simulink model "Simulacion_Estrategias"  (R2016a)
settings: Solver=VariableStepAuto  StartTime=0.0  StopTime=5  RelTol=1e-3
undefined symbols (not defined in the file): AL, BL, CL, DL, Kes_PC, Kest_LQR, Ki_PC, u10, u20, u30, x10, x20, x30, xini1
libraries: cstblocks x12
settings Model: Creator=Lenovo  LastModifiedBy=Lenovo

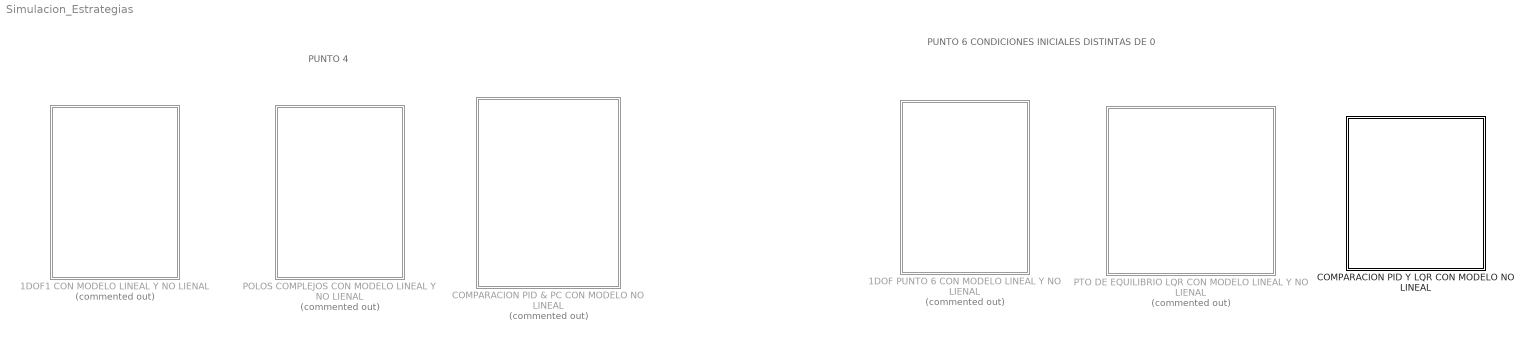
== system Simulacion_Estrategias ==
  note: PUNTO 6 CONDICIONES INICIALES DISTINTAS DE 0
  note: PUNTO 4
  1DOF PUNTO 6 CON MODELO LINEAL Y NO LIENAL : Subsystem  Commented=on
  1DOF1 CON MODELO LINEAL Y NO LIENAL : Subsystem  Commented=on
  COMPARACION PID & PC CON MODELO NO LINEAL : Subsystem  Commented=on
  COMPARACION PID Y LQR CON MODELO NO LINEAL : Subsystem
  "POLOS COMPLEJOS CON MODELO LINEAL Y NO LIENAL " : Subsystem  Commented=on
  PTO DE EQUILIBRIO LQR CON MODELO LINEAL Y NO LIENAL : Subsystem  Commented=on

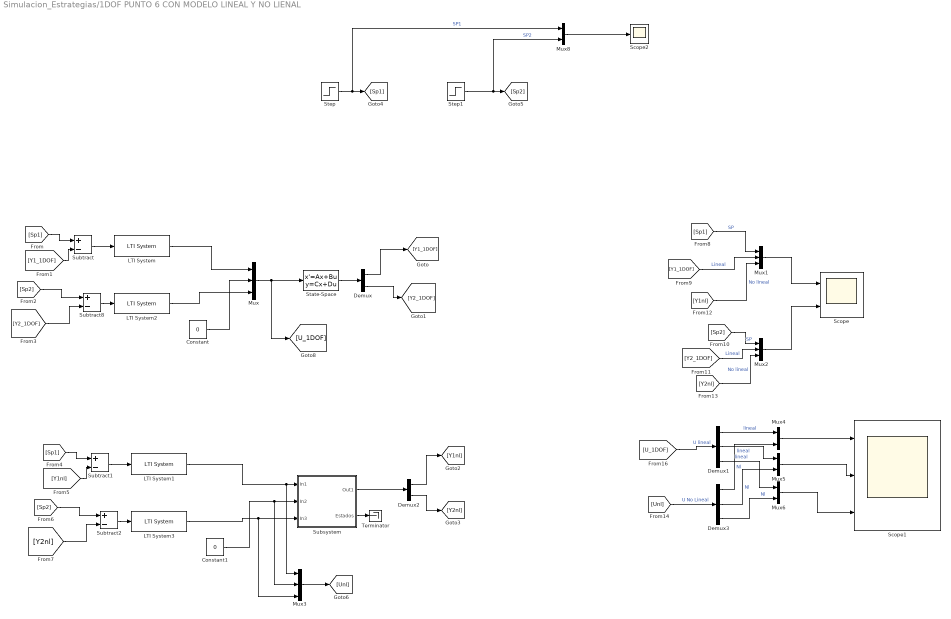
== system Simulacion_Estrategias/1DOF PUNTO 6 CON MODELO LINEAL Y NO LIENAL ==
  Constant : Constant  Value=0
  Constant1 : Constant  Value=0
  Demux : Demux  Outputs=2
  Demux1 : Demux  Outputs=3
  Demux2 : Demux  Outputs=2
  Demux3 : Demux  Outputs=3
  LTI System : cstblocks/LTI System  sys=C11  IC=[]
  LTI System1 : cstblocks/LTI System  sys=C11  IC=[]
  LTI System2 : cstblocks/LTI System  sys=C23  IC=[]
  LTI System3 : cstblocks/LTI System  sys=C23  IC=[]
  Mux{,1..3} (4 alike) : Mux  Inputs=3
  Mux{4..6,8} (4 alike) : Mux  Inputs=2
  Scope : Scope  NumInputPorts=2
  Scope1 : Scope  NumInputPorts=3
  Scope2 : Scope
  State-Space : StateSpace  A=AL  B=BL  C=CL  D=DL  X0=xini1
  Step : Step  Time=0  After=0  SampleTime=0
  Step1 : Step  Time=0  After=0  SampleTime=0
  Subsystem : Subsystem
  Subtract{,1..2,8} (4 alike) : Sum  Inputs=+-
  Terminator : Terminator
  wires:
  Constant1/1 -> Subsystem/2(In2), Mux3/2
  LTI System3/1 -> Subsystem/3(In3), Mux3/3
  LTI System1/1 -> Subsystem/1(In1), Mux3/1
  LTI System2/1 -> Mux/3
  Constant/1 -> Mux/2
  LTI System/1 -> Mux/1
  [Y1nl] -> Subtract1/2
  [Sp1] -> Subtract1/1
  [Sp2] -> Subtract2/1
  Subtract2/1 -> LTI System3/1
  Subtract1/1 -> LTI System1/1
  [Y2nl] -> Subtract2/2
  Demux3/3 -> Mux6/2  "Nl"
  Demux3/2 -> Mux5/2  "Nl"
  Demux3/1 -> Mux4/2  "Nl"
  Demux1/3 -> Mux6/1  "lineal"
  Demux1/2 -> Mux5/1  "lineal"
  Demux1/1 -> Mux4/1  "lineal"
  Mux6/1 -> Scope1/3
  [Y2nl] -> Mux2/3  "No lineal"
  [Y1_1DOF] -> Mux1/2  "Lineal"
  [U_1DOF] -> Demux1/1  "U lineal"
  Mux5/1 -> Scope1/2
  [Unl] -> Demux3/1  "U No Lineal"
  Demux2/1 -> [Y1nl]
  [Y1nl] -> Mux1/3  "No lineal"
  [Sp1] -> Mux1/1  "SP"
  Mux2/1 -> Scope/2
  Mux4/1 -> Scope1/1
  [Sp2] -> Mux2/1  "SP"
  Subsystem/1(Out1) -> Demux2/1
  Demux2/2 -> [Y2nl]
  Mux1/1 -> Scope/1
  [Y2_1DOF] -> Mux2/2  "Lineal"
  State-Space/1 -> Demux/1
  [Y2_1DOF] -> Subtract8/2
  Subtract/1 -> LTI System/1
  Subtract8/1 -> LTI System2/1
  [Sp2] -> Subtract8/1
  Mux/1 -> [U_1DOF], State-Space/1
  Demux/2 -> [Y2_1DOF]
  Demux/1 -> [Y1_1DOF]
  [Sp1] -> Subtract/1
  [Y1_1DOF] -> Subtract/2
  Mux3/1 -> [Unl]
  Subsystem/2(Estados) -> Terminator/1
  Step/1 -> Mux8/1, [Sp1]  "SP1"
  Step1/1 -> Mux8/2, [Sp2]  "SP2"
  Mux8/1 -> Scope2/1

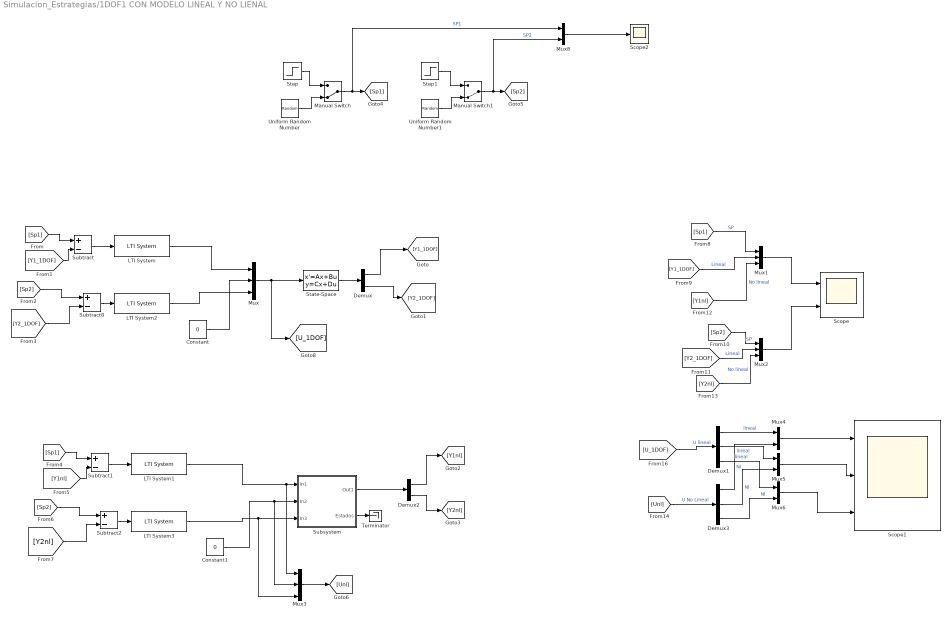
== system Simulacion_Estrategias/1DOF1 CON MODELO LINEAL Y NO LIENAL ==
  Constant : Constant  Value=0
  Constant1 : Constant  Value=0
  Demux : Demux  Outputs=2
  Demux1 : Demux  Outputs=3
  Demux2 : Demux  Outputs=2
  Demux3 : Demux  Outputs=3
  LTI System : cstblocks/LTI System  sys=C11  IC=[]
  LTI System1 : cstblocks/LTI System  sys=C11  IC=[]
  LTI System2 : cstblocks/LTI System  sys=C23  IC=[]
  LTI System3 : cstblocks/LTI System  sys=C23  IC=[]
  Manual Switch : ManualSwitch  CurrentSetting=0
  Manual Switch1 : ManualSwitch  CurrentSetting=0
  Mux{,1..3} (4 alike) : Mux  Inputs=3
  Mux{4..6,8} (4 alike) : Mux  Inputs=2
  Scope : Scope  NumInputPorts=2
  Scope1 : Scope  NumInputPorts=3
  Scope2 : Scope
  State-Space : StateSpace  A=AL  B=BL  C=CL  D=DL
  Step : Step  Time=0  SampleTime=0
  Step1 : Step  Time=0  After=0  SampleTime=0
  Subsystem : Subsystem
  Subtract{,1..2,8} (4 alike) : Sum  Inputs=+-
  Terminator : Terminator
  Uniform Random Number : UniformRandomNumber  Minimum=-0-5  Maximum=0.5  SampleTime=4
  Uniform Random Number1 : UniformRandomNumber  Minimum=-0.5  Maximum=0.5  SampleTime=7
  wires:
  Mux8/1 -> Scope2/1
  Manual Switch1/1 -> [Sp2], Mux8/2  "SP2"
  Step1/1 -> Manual Switch1/1
  Uniform Random Number/1 -> Manual Switch/2
  Manual Switch/1 -> [Sp1], Mux8/1  "SP1"
  Step/1 -> Manual Switch/1
  Uniform Random Number1/1 -> Manual Switch1/2
  Subsystem/2(Estados) -> Terminator/1
  Mux3/1 -> [Unl]
  [Y1_1DOF] -> Subtract/2
  [Sp1] -> Subtract/1
  Demux/1 -> [Y1_1DOF]
  Demux/2 -> [Y2_1DOF]
  Mux/1 -> State-Space/1, [U_1DOF]
  [Sp2] -> Subtract8/1
  Subtract8/1 -> LTI System2/1
  Subtract/1 -> LTI System/1
  [Y2_1DOF] -> Subtract8/2
  State-Space/1 -> Demux/1
  [Y2_1DOF] -> Mux2/2  "Lineal"
  Mux1/1 -> Scope/1
  Demux2/2 -> [Y2nl]
  Subsystem/1(Out1) -> Demux2/1
  [Sp2] -> Mux2/1  "SP"
  Mux4/1 -> Scope1/1
  Mux2/1 -> Scope/2
  [Sp1] -> Mux1/1  "SP"
  [Y1nl] -> Mux1/3  "No lineal"
  Demux2/1 -> [Y1nl]
  [Unl] -> Demux3/1  "U No Lineal"
  Mux5/1 -> Scope1/2
  [U_1DOF] -> Demux1/1  "U lineal"
  [Y1_1DOF] -> Mux1/2  "Lineal"
  [Y2nl] -> Mux2/3  "No lineal"
  Mux6/1 -> Scope1/3
  Demux1/1 -> Mux4/1  "lineal"
  Demux1/2 -> Mux5/1  "lineal"
  Demux1/3 -> Mux6/1  "lineal"
  Demux3/1 -> Mux4/2  "Nl"
  Demux3/2 -> Mux5/2  "Nl"
  Demux3/3 -> Mux6/2  "Nl"
  [Y2nl] -> Subtract2/2
  Subtract1/1 -> LTI System1/1
  Subtract2/1 -> LTI System3/1
  [Sp2] -> Subtract2/1
  [Sp1] -> Subtract1/1
  [Y1nl] -> Subtract1/2
  LTI System/1 -> Mux/1
  Constant/1 -> Mux/2
  LTI System2/1 -> Mux/3
  LTI System1/1 -> Mux3/1, Subsystem/1(In1)
  LTI System3/1 -> Mux3/3, Subsystem/3(In3)
  Constant1/1 -> Mux3/2, Subsystem/2(In2)

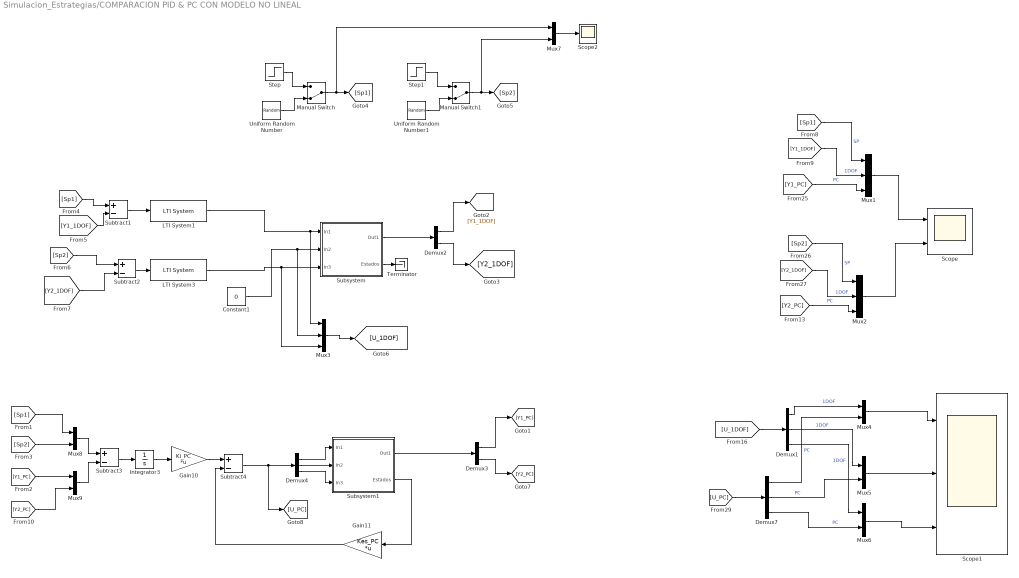
== system Simulacion_Estrategias/COMPARACION PID & PC CON MODELO NO LINEAL ==
  Constant1 : Constant  Value=0
  Demux1 : Demux  Outputs=3
  Demux2 : Demux  Outputs=2
  Demux3 : Demux  Outputs=2
  Demux4 : Demux  Outputs=3
  Demux7 : Demux  Outputs=3
  Gain10 : Gain  Gain=Ki_PC  Multiplication=Matrix(K*u)
  Gain11 : Gain  Gain=Kes_PC  Multiplication=Matrix(K*u)
  Integrator3 : Integrator
  LTI System1 : cstblocks/LTI System  sys=C11  IC=[]
  LTI System3 : cstblocks/LTI System  sys=C23  IC=[]
  Manual Switch : ManualSwitch  CurrentSetting=0
  Manual Switch1 : ManualSwitch  CurrentSetting=0
  Mux1 : Mux  Inputs=3
  Mux2 : Mux  Inputs=3
  Mux3 : Mux  Inputs=3
  Mux{4..9} (6 alike) : Mux  Inputs=2
  Scope : Scope  NumInputPorts=2
  Scope1 : Scope  NumInputPorts=3
  Scope2 : Scope
  Step : Step  Time=0  After=0  SampleTime=0
  Step1 : Step  Time=0  SampleTime=0
  Subsystem : Subsystem
  Subsystem1 : Subsystem
  Subtract{1..4} (4 alike) : Sum  Inputs=+-
  Terminator : Terminator
  Uniform Random Number : UniformRandomNumber  Minimum=-0.5  Maximum=0.5  SampleTime=6
  Uniform Random Number1 : UniformRandomNumber  Minimum=-0.5  Maximum=0.5  SampleTime=9
  wires:
  Uniform Random Number1/1 -> Manual Switch1/2
  Mux7/1 -> Scope2/1
  Manual Switch1/1 -> [Sp2], Mux7/2
  Uniform Random Number/1 -> Manual Switch/2
  Manual Switch/1 -> [Sp1], Mux7/1
  Step/1 -> Manual Switch/1
  Step1/1 -> Manual Switch1/1
  Mux5/1 -> Scope1/2
  Mux6/1 -> Scope1/3
  [Sp1] -> Mux1/1  "SP"
  [Y1_1DOF] -> Mux1/2  "1DOF"
  Mux1/1 -> Scope/1
  [U_PC] -> Demux7/1
  [U_1DOF] -> Demux1/1
  Demux1/3 -> Mux6/1  "1DOF"
  [Y2_1DOF] -> Mux2/2  "1DOF"
  [Y1_PC] -> Mux1/3  "PC"
  Demux1/2 -> Mux5/1  "1DOF"
  Mux4/1 -> Scope1/1
  Demux1/1 -> Mux4/1  "1DOF"
  Mux2/1 -> Scope/2
  [Sp2] -> Mux2/1  "SP"
  [Y2_PC] -> Mux2/3  "PC"
  Demux7/1 -> Mux4/2  "PC"
  Demux7/2 -> Mux5/2  "PC"
  Demux7/3 -> Mux6/2  "PC"
  LTI System1/1 -> Mux3/1, Subsystem/1(In1)
  Subtract2/1 -> LTI System3/1
  [Sp1] -> Subtract1/1
  [Y1_1DOF] -> Subtract1/2
  [Y2_1DOF] -> Subtract2/2
  Subsystem/2(Estados) -> Terminator/1
  [Sp2] -> Subtract2/1
  Demux2/1 -> [Y1_1DOF]
  Mux3/1 -> [U_1DOF]
  Subsystem/1(Out1) -> Demux2/1
  Subtract1/1 -> LTI System1/1
  Demux2/2 -> [Y2_1DOF]
  Constant1/1 -> Mux3/2, Subsystem/2(In2)
  LTI System3/1 -> Mux3/3, Subsystem/3(In3)
  Subsystem1/2(Estados) -> Gain11/1
  Demux4/2 -> Subsystem1/2(In2)
  Subsystem1/1(Out1) -> Demux3/1
  Demux4/1 -> Subsystem1/1(In1)
  [Y1_PC] -> Mux9/1
  Mux8/1 -> Subtract3/1
  Demux4/3 -> Subsystem1/3(In3)
  Subtract3/1 -> Integrator3/1
  Gain10/1 -> Subtract4/1
  [Sp2] -> Mux8/2
  Gain11/1 -> Subtract4/2
  Integrator3/1 -> Gain10/1
  Subtract4/1 -> [U_PC], Demux4/1
  [Sp1] -> Mux8/1
  [Y2_PC] -> Mux9/2
  Demux3/2 -> [Y2_PC]
  Mux9/1 -> Subtract3/2
  Demux3/1 -> [Y1_PC]

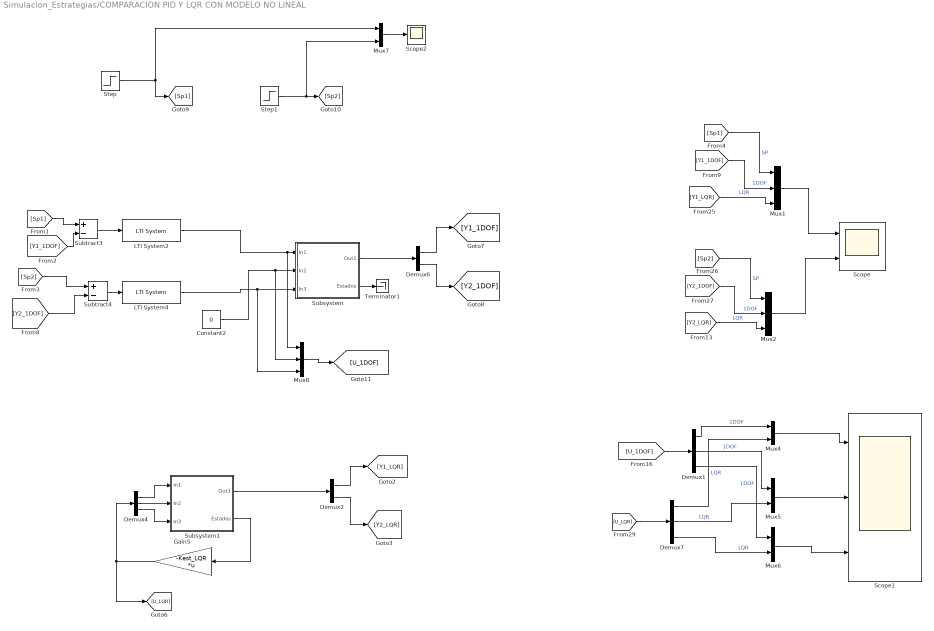
== system Simulacion_Estrategias/COMPARACION PID Y LQR CON MODELO NO LINEAL ==
  Constant2 : Constant  Value=0
  Demux1 : Demux  Outputs=3
  Demux2 : Demux  Outputs=2
  Demux4 : Demux  Outputs=3
  Demux6 : Demux  Outputs=2
  Demux7 : Demux  Outputs=3
  Gain5 : Gain  Gain=-Kest_LQR  Multiplication=Matrix(K*u)
  LTI System2 : cstblocks/LTI System  sys=C11  IC=[]
  LTI System4 : cstblocks/LTI System  sys=C23  IC=[]
  Mux1 : Mux  Inputs=3
  Mux2 : Mux  Inputs=3
  Mux{4..7} (4 alike) : Mux  Inputs=2
  Mux8 : Mux  Inputs=3
  Scope : Scope  NumInputPorts=2
  Scope1 : Scope  NumInputPorts=3
  Scope2 : Scope
  Step : Step  Time=0  After=0  SampleTime=0
  Step1 : Step  Time=0  After=0  SampleTime=0
  Subsystem : Subsystem
  Subsystem1 : Subsystem
  Subtract3 : Sum  Inputs=+-
  Subtract4 : Sum  Inputs=+-
  Terminator1 : Terminator
  wires:
  Step/1 -> [Sp1], Mux7/1
  Mux7/1 -> Scope2/1
  Step1/1 -> [Sp2], Mux7/2
  Demux4/1 -> Subsystem1/1(In1)
  Subsystem1/2(Estados) -> Gain5/1
  Subsystem1/1(Out1) -> Demux2/1
  Gain5/1 -> Demux4/1, [U_LQR]
  Demux4/2 -> Subsystem1/2(In2)
  Demux2/1 -> [Y1_LQR]
  Demux2/2 -> [Y2_LQR]
  Demux4/3 -> Subsystem1/3(In3)
  LTI System4/1 -> Subsystem/3(In3), Mux8/3
  Subtract3/1 -> LTI System2/1
  Constant2/1 -> Subsystem/2(In2), Mux8/2
  Demux6/2 -> [Y2_1DOF]
  Subsystem/1(Out1) -> Demux6/1
  Mux8/1 -> [U_1DOF]
  [Sp1] -> Subtract3/1
  Subsystem/2(Estados) -> Terminator1/1
  [Y2_1DOF] -> Subtract4/2
  Demux6/1 -> [Y1_1DOF]
  [Y1_1DOF] -> Subtract3/2
  Subtract4/1 -> LTI System4/1
  [Sp2] -> Subtract4/1
  LTI System2/1 -> Subsystem/1(In1), Mux8/1
  [Sp2] -> Mux2/1  "SP"
  Mux2/1 -> Scope/2
  Demux7/1 -> Mux4/2  "LQR"
  [U_LQR] -> Demux7/1
  Demux1/3 -> Mux6/1  "1DOF"
  [Y2_LQR] -> Mux2/3  "LQR"
  Demux7/2 -> Mux5/2  "LQR"
  Mux4/1 -> Scope1/1
  [Y2_1DOF] -> Mux2/2  "1DOF"
  [Y1_LQR] -> Mux1/3  "LQR"
  Demux1/2 -> Mux5/1  "1DOF"
  [U_1DOF] -> Demux1/1
  Demux1/1 -> Mux4/1  "1DOF"
  Mux1/1 -> Scope/1
  Mux5/1 -> Scope1/2
  Mux6/1 -> Scope1/3
  Demux7/3 -> Mux6/2  "LQR"
  [Y1_1DOF] -> Mux1/2  "1DOF"
  [Sp1] -> Mux1/1  "SP"

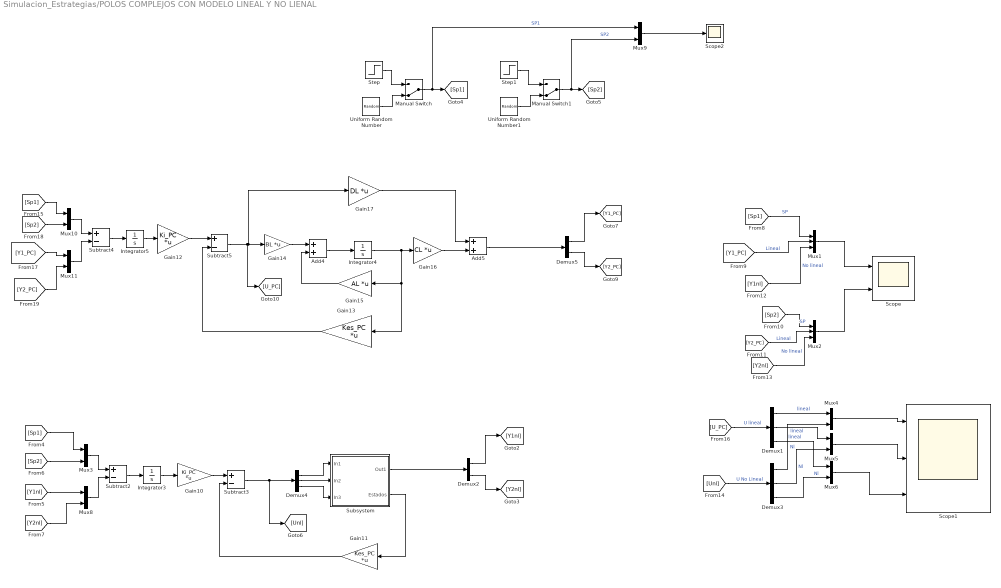
== system Simulacion_Estrategias/POLOS COMPLEJOS CON MODELO LINEAL Y NO LIENAL  ==
  Add4 : Sum
  Add5 : Sum
  Demux1 : Demux  Outputs=3
  Demux2 : Demux  Outputs=2
  Demux3 : Demux  Outputs=3
  Demux4 : Demux  Outputs=3
  Demux5 : Demux  Outputs=2
  Gain10 : Gain  Gain=Ki_PC  Multiplication=Matrix(K*u)
  Gain11 : Gain  Gain=Kes_PC  Multiplication=Matrix(K*u)
  Gain12 : Gain  Gain=Ki_PC  Multiplication=Matrix(K*u)
  Gain13 : Gain  Gain=Kes_PC  Multiplication=Matrix(K*u)
  Gain14 : Gain  Gain=BL  Multiplication=Matrix(K*u)
  Gain15 : Gain  Gain=AL  Multiplication=Matrix(K*u)
  Gain16 : Gain  Gain=CL  Multiplication=Matrix(K*u)
  Gain17 : Gain  Gain=DL  Multiplication=Matrix(K*u)
  Integrator3 : Integrator
  Integrator4 : Integrator
  Integrator5 : Integrator
  Manual Switch : ManualSwitch  CurrentSetting=0
  Manual Switch1 : ManualSwitch  CurrentSetting=0
  Mux1 : Mux  Inputs=3
  Mux{3..6,8..11} (8 alike) : Mux  Inputs=2
  Mux2 : Mux  Inputs=3
  Scope : Scope  NumInputPorts=2
  Scope1 : Scope  NumInputPorts=3
  Scope2 : Scope
  Step : Step  Time=0  SampleTime=0
  Step1 : Step  Time=0  After=0  SampleTime=0
  Subsystem : Subsystem
  Subtract{2..5} (4 alike) : Sum  Inputs=+-
  Uniform Random Number : UniformRandomNumber  Minimum=-0.5  Maximum=0.5  SampleTime=6
  Uniform Random Number1 : UniformRandomNumber  Minimum=-0.5  Maximum=0.5  SampleTime=10
  wires:
  Gain11/1 -> Subtract3/2
  [Y2_PC] -> Mux2/2  "Lineal"
  Mux1/1 -> Scope/1
  Demux2/2 -> [Y2nl]
  [Sp1] -> Mux3/1
  Mux3/1 -> Subtract2/1
  [Sp2] -> Mux2/1  "SP"
  Demux4/2 -> Subsystem/2(In2)
  Mux4/1 -> Scope1/1
  Mux2/1 -> Scope/2
  [Sp2] -> Mux3/2
  [Sp1] -> Mux1/1  "SP"
  Mux8/1 -> Subtract2/2
  [Y1nl] -> Mux1/3  "No lineal"
  [Y2nl] -> Mux8/2
  Subtract3/1 -> [Unl], Demux4/1
  Integrator3/1 -> Gain10/1
  Demux2/1 -> [Y1nl]
  [Unl] -> Demux3/1  "U No Lineal"
  Subsystem/2(Estados) -> Gain11/1
  Mux5/1 -> Scope1/2
  [U_PC] -> Demux1/1  "U lineal"
  [Y1_PC] -> Mux1/2  "Lineal"
  [Y2nl] -> Mux2/3  "No lineal"
  [Y1nl] -> Mux8/1
  Gain10/1 -> Subtract3/1
  Subtract2/1 -> Integrator3/1
  Gain12/1 -> Subtract5/1
  Subtract4/1 -> Integrator5/1
  Subtract5/1 -> Gain14/1, Gain17/1, [U_PC]
  Integrator4/1 -> Gain16/1, Gain15/1, Gain13/1
  Demux5/1 -> [Y1_PC]
  Gain15/1 -> Add4/2
  Add5/1 -> Demux5/1
  Mux11/1 -> Subtract4/2
  Mux10/1 -> Subtract4/1
  Demux5/2 -> [Y2_PC]
  Gain17/1 -> Add5/1
  Gain13/1 -> Subtract5/2
  [Sp1] -> Mux10/1
  Gain16/1 -> Add5/2
  [Sp2] -> Mux10/2
  [Y1_PC] -> Mux11/1
  [Y2_PC] -> Mux11/2
  Add4/1 -> Integrator4/1
  Integrator5/1 -> Gain12/1
  Gain14/1 -> Add4/1
  Mux6/1 -> Scope1/3
  Demux1/1 -> Mux4/1  "lineal"
  Demux1/2 -> Mux5/1  "lineal"
  Demux1/3 -> Mux6/1  "lineal"
  Demux3/1 -> Mux4/2  "Nl"
  Demux3/2 -> Mux5/2  "Nl"
  Demux3/3 -> Mux6/2  "Nl"
  Demux4/1 -> Subsystem/1(In1)
  Demux4/3 -> Subsystem/3(In3)
  Subsystem/1(Out1) -> Demux2/1
  Manual Switch1/1 -> [Sp2], Mux9/2  "SP2"
  Uniform Random Number/1 -> Manual Switch/2
  Manual Switch/1 -> [Sp1], Mux9/1  "SP1"
  Step/1 -> Manual Switch/1
  Uniform Random Number1/1 -> Manual Switch1/2
  Step1/1 -> Manual Switch1/1
  Mux9/1 -> Scope2/1

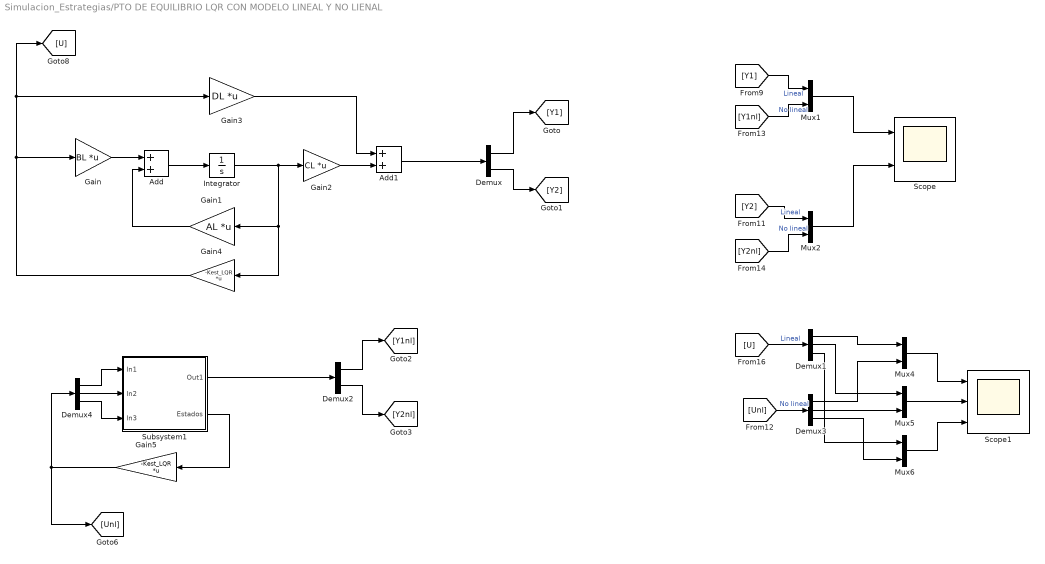
== system Simulacion_Estrategias/PTO DE EQUILIBRIO LQR CON MODELO LINEAL Y NO LIENAL ==
  Add : Sum
  Add1 : Sum
  Demux : Demux  Outputs=2
  Demux1 : Demux  Outputs=3
  Demux2 : Demux  Outputs=2
  Demux3 : Demux  Outputs=3
  Demux4 : Demux  Outputs=3
  Gain : Gain  Gain=BL  Multiplication=Matrix(K*u)
  Gain1 : Gain  Gain=AL  Multiplication=Matrix(K*u)
  Gain2 : Gain  Gain=CL  Multiplication=Matrix(K*u)
  Gain3 : Gain  Gain=DL  Multiplication=Matrix(K*u)
  Gain4 : Gain  Gain=-Kest_LQR  Multiplication=Matrix(K*u)
  Gain5 : Gain  Gain=-Kest_LQR  Multiplication=Matrix(K*u)
  Integrator : Integrator  InitialCondition=xini1
  Mux{1..2,4..6} (5 alike) : Mux  Inputs=2
  Scope : Scope  NumInputPorts=2
  Scope1 : Scope  NumInputPorts=3
  Subsystem1 : Subsystem
  wires:
  Demux/2 -> [Y2]
  Mux1/1 -> Scope/1
  Integrator/1 -> Gain4/1, Gain1/1, Gain2/1
  Gain3/1 -> Add1/1
  Gain/1 -> Add/1
  Demux1/2 -> Mux5/1
  [Y2nl] -> Mux2/2  "No lineal"
  Gain4/1 -> [U], Gain3/1, Gain/1
  Demux4/2 -> Subsystem1/2(In2)
  Mux2/1 -> Scope/2
  Gain5/1 -> Demux4/1, [Unl]
  Add1/1 -> Demux/1
  [U] -> Demux1/1  "Lineal"
  Demux1/1 -> Mux4/1
  Demux2/2 -> [Y2nl]
  Gain2/1 -> Add1/2
  Add/1 -> Integrator/1
  Demux3/1 -> Mux4/2
  Mux6/1 -> Scope1/3
  Demux4/3 -> Subsystem1/3(In3)
  Demux4/1 -> Subsystem1/1(In1)
  Demux3/2 -> Mux5/2
  [Y1] -> Mux1/1  "Lineal"
  Mux5/1 -> Scope1/2
  Gain1/1 -> Add/2
  Mux4/1 -> Scope1/1
  [Unl] -> Demux3/1  "No lineal"
  [Y2] -> Mux2/1  "Lineal"
  Demux1/3 -> Mux6/1
  Demux2/1 -> [Y1nl]
  Subsystem1/1(Out1) -> Demux2/1
  [Y1nl] -> Mux1/2  "No lineal"
  Subsystem1/2(Estados) -> Gain5/1
  Demux3/3 -> Mux6/2
  Demux/1 -> [Y1]

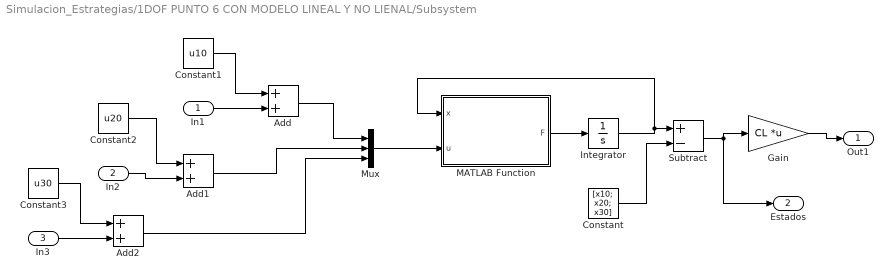
== system Simulacion_Estrategias/1DOF PUNTO 6 CON MODELO LINEAL Y NO LIENAL/Subsystem ==
  In1 : Inport
  In2 : Inport  Port=2
  In3 : Inport  Port=3
  Add : Sum
  Add1 : Sum
  Add2 : Sum
  Constant : Constant  Value=[x10; x20; x30]
  Constant1 : Constant  Value=u10
  Constant2 : Constant  Value=u20
  Constant3 : Constant  Value=u30
  Gain : Gain  Gain=CL  Multiplication=Matrix(K*u)
  Integrator : Integrator  InitialCondition=[x10; x20; x30]+xini1
  MATLAB Function : MATLAB Function  TreatAsAtomicUnit=on
  Mux : Mux  Inputs=3
  Subtract : Sum  Inputs=+-
  Out1 : Outport
  Estados : Outport  Port=2
  wires:
  Mux/1 -> MATLAB Function/2(u)
  Add2/1 -> Mux/3
  In3/1 -> Add2/2
  Constant3/1 -> Add2/1
  Add1/1 -> Mux/2
  In2/1 -> Add1/2
  Constant2/1 -> Add1/1
  Constant1/1 -> Add/1
  In1/1 -> Add/2
  Add/1 -> Mux/1
  MATLAB Function/1(F) -> Integrator/1
  Gain/1 -> Out1/1
  Subtract/1 -> Gain/1, Estados/1
  Constant/1 -> Subtract/2
  Integrator/1 -> Subtract/1, MATLAB Function/1(x)

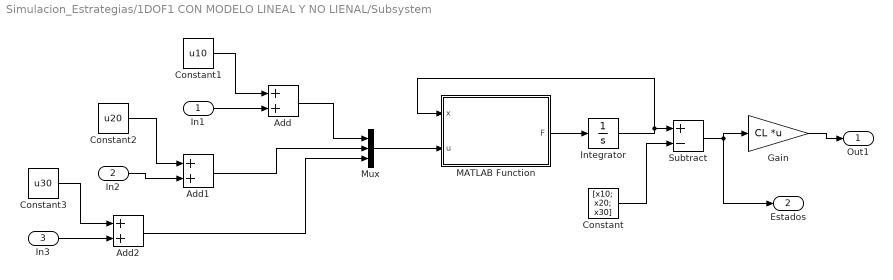
== system Simulacion_Estrategias/1DOF1 CON MODELO LINEAL Y NO LIENAL/Subsystem ==
  In1 : Inport
  In2 : Inport  Port=2
  In3 : Inport  Port=3
  Add : Sum
  Add1 : Sum
  Add2 : Sum
  Constant : Constant  Value=[x10; x20; x30]
  Constant1 : Constant  Value=u10
  Constant2 : Constant  Value=u20
  Constant3 : Constant  Value=u30
  Gain : Gain  Gain=CL  Multiplication=Matrix(K*u)
  Integrator : Integrator  InitialCondition=[x10; x20; x30]
  MATLAB Function : MATLAB Function  TreatAsAtomicUnit=on
  Mux : Mux  Inputs=3
  Subtract : Sum  Inputs=+-
  Out1 : Outport
  Estados : Outport  Port=2
  wires:
  Integrator/1 -> MATLAB Function/1(x), Subtract/1
  Constant/1 -> Subtract/2
  Subtract/1 -> Estados/1, Gain/1
  Gain/1 -> Out1/1
  MATLAB Function/1(F) -> Integrator/1
  Add/1 -> Mux/1
  In1/1 -> Add/2
  Constant1/1 -> Add/1
  Constant2/1 -> Add1/1
  In2/1 -> Add1/2
  Add1/1 -> Mux/2
  Constant3/1 -> Add2/1
  In3/1 -> Add2/2
  Add2/1 -> Mux/3
  Mux/1 -> MATLAB Function/2(u)

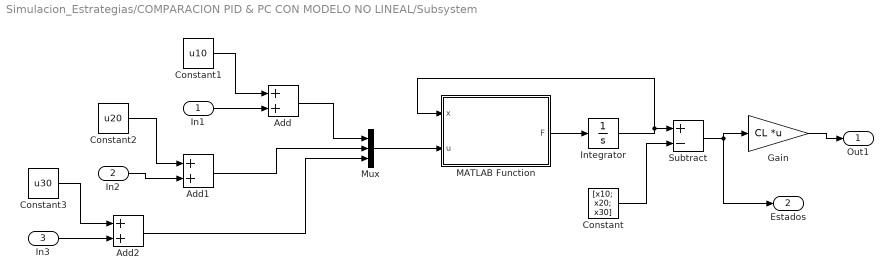
== system Simulacion_Estrategias/COMPARACION PID & PC CON MODELO NO LINEAL/Subsystem ==
  In1 : Inport
  In2 : Inport  Port=2
  In3 : Inport  Port=3
  Add : Sum
  Add1 : Sum
  Add2 : Sum
  Constant : Constant  Value=[x10; x20; x30]
  Constant1 : Constant  Value=u10
  Constant2 : Constant  Value=u20
  Constant3 : Constant  Value=u30
  Gain : Gain  Gain=CL  Multiplication=Matrix(K*u)
  Integrator : Integrator  InitialCondition=[x10; x20; x30]
  MATLAB Function : MATLAB Function  TreatAsAtomicUnit=on
  Mux : Mux  Inputs=3
  Subtract : Sum  Inputs=+-
  Out1 : Outport
  Estados : Outport  Port=2
  wires:
  Integrator/1 -> MATLAB Function/1(x), Subtract/1
  Constant/1 -> Subtract/2
  Subtract/1 -> Estados/1, Gain/1
  Gain/1 -> Out1/1
  MATLAB Function/1(F) -> Integrator/1
  Add/1 -> Mux/1
  In1/1 -> Add/2
  Constant1/1 -> Add/1
  Constant2/1 -> Add1/1
  In2/1 -> Add1/2
  Add1/1 -> Mux/2
  Constant3/1 -> Add2/1
  In3/1 -> Add2/2
  Add2/1 -> Mux/3
  Mux/1 -> MATLAB Function/2(u)

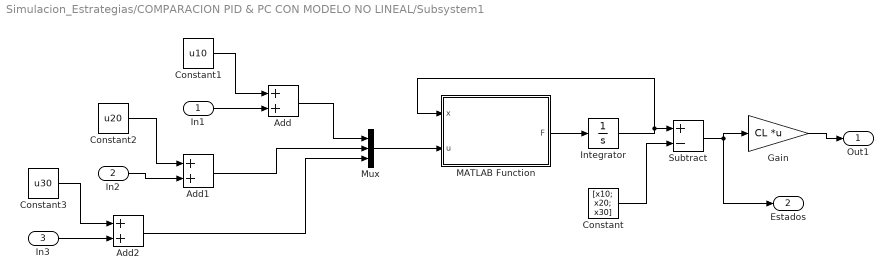
== system Simulacion_Estrategias/COMPARACION PID & PC CON MODELO NO LINEAL/Subsystem1 ==
  In1 : Inport
  In2 : Inport  Port=2
  In3 : Inport  Port=3
  Add : Sum
  Add1 : Sum
  Add2 : Sum
  Constant : Constant  Value=[x10; x20; x30]
  Constant1 : Constant  Value=u10
  Constant2 : Constant  Value=u20
  Constant3 : Constant  Value=u30
  Gain : Gain  Gain=CL  Multiplication=Matrix(K*u)
  Integrator : Integrator  InitialCondition=[x10; x20; x30]
  MATLAB Function : MATLAB Function  TreatAsAtomicUnit=on
  Mux : Mux  Inputs=3
  Subtract : Sum  Inputs=+-
  Out1 : Outport
  Estados : Outport  Port=2
  wires:
  Integrator/1 -> MATLAB Function/1(x), Subtract/1
  Constant/1 -> Subtract/2
  Subtract/1 -> Estados/1, Gain/1
  Gain/1 -> Out1/1
  MATLAB Function/1(F) -> Integrator/1
  Add/1 -> Mux/1
  In1/1 -> Add/2
  Constant1/1 -> Add/1
  Constant2/1 -> Add1/1
  In2/1 -> Add1/2
  Add1/1 -> Mux/2
  Constant3/1 -> Add2/1
  In3/1 -> Add2/2
  Add2/1 -> Mux/3
  Mux/1 -> MATLAB Function/2(u)

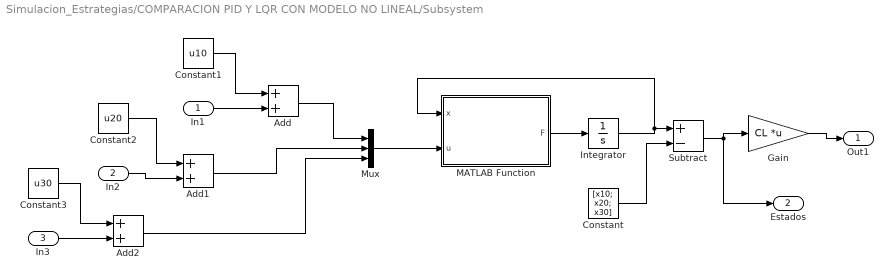
== system Simulacion_Estrategias/COMPARACION PID Y LQR CON MODELO NO LINEAL/Subsystem ==
  In1 : Inport
  In2 : Inport  Port=2
  In3 : Inport  Port=3
  Add : Sum
  Add1 : Sum
  Add2 : Sum
  Constant : Constant  Value=[x10; x20; x30]
  Constant1 : Constant  Value=u10
  Constant2 : Constant  Value=u20
  Constant3 : Constant  Value=u30
  Gain : Gain  Gain=CL  Multiplication=Matrix(K*u)
  Integrator : Integrator  InitialCondition=[x10; x20; x30]+xini1
  MATLAB Function : MATLAB Function  TreatAsAtomicUnit=on
  Mux : Mux  Inputs=3
  Subtract : Sum  Inputs=+-
  Out1 : Outport
  Estados : Outport  Port=2
  wires:
  Mux/1 -> MATLAB Function/2(u)
  Add2/1 -> Mux/3
  In3/1 -> Add2/2
  Constant3/1 -> Add2/1
  Add1/1 -> Mux/2
  In2/1 -> Add1/2
  Constant2/1 -> Add1/1
  Constant1/1 -> Add/1
  In1/1 -> Add/2
  Add/1 -> Mux/1
  MATLAB Function/1(F) -> Integrator/1
  Gain/1 -> Out1/1
  Subtract/1 -> Gain/1, Estados/1
  Constant/1 -> Subtract/2
  Integrator/1 -> Subtract/1, MATLAB Function/1(x)

== system Simulacion_Estrategias/COMPARACION PID Y LQR CON MODELO NO LINEAL/Subsystem1 ==
  In1 : Inport
  In2 : Inport  Port=2
  In3 : Inport  Port=3
  Add : Sum
  Add1 : Sum
  Add2 : Sum
  Constant : Constant  Value=[x10; x20; x30]
  Constant1 : Constant  Value=u10
  Constant2 : Constant  Value=u20
  Constant3 : Constant  Value=u30
  Gain : Gain  Gain=CL  Multiplication=Matrix(K*u)
  Integrator : Integrator  InitialCondition=[x10; x20; x30]+xini1
  MATLAB Function : MATLAB Function  TreatAsAtomicUnit=on
  Mux : Mux  Inputs=3
  Subtract : Sum  Inputs=+-
  Out1 : Outport
  Estados : Outport  Port=2
  wires:
  Mux/1 -> MATLAB Function/2(u)
  Add2/1 -> Mux/3
  In3/1 -> Add2/2
  Constant3/1 -> Add2/1
  Add1/1 -> Mux/2
  In2/1 -> Add1/2
  Constant2/1 -> Add1/1
  Constant1/1 -> Add/1
  In1/1 -> Add/2
  Add/1 -> Mux/1
  MATLAB Function/1(F) -> Integrator/1
  Gain/1 -> Out1/1
  Subtract/1 -> Gain/1, Estados/1
  Constant/1 -> Subtract/2
  Integrator/1 -> Subtract/1, MATLAB Function/1(x)

== system Simulacion_Estrategias/POLOS COMPLEJOS CON MODELO LINEAL Y NO LIENAL /Subsystem ==
  In1 : Inport
  In2 : Inport  Port=2
  In3 : Inport  Port=3
  Add : Sum
  Add1 : Sum
  Add2 : Sum
  Constant : Constant  Value=[x10; x20; x30]
  Constant1 : Constant  Value=u10
  Constant2 : Constant  Value=u20
  Constant3 : Constant  Value=u30
  Gain : Gain  Gain=CL  Multiplication=Matrix(K*u)
  Integrator : Integrator  InitialCondition=[x10; x20; x30]
  MATLAB Function : MATLAB Function  TreatAsAtomicUnit=on
  Mux : Mux  Inputs=3
  Subtract : Sum  Inputs=+-
  Out1 : Outport
  Estados : Outport  Port=2
  wires:
  Integrator/1 -> MATLAB Function/1(x), Subtract/1
  Constant/1 -> Subtract/2
  Subtract/1 -> Estados/1, Gain/1
  Gain/1 -> Out1/1
  MATLAB Function/1(F) -> Integrator/1
  Add/1 -> Mux/1
  In1/1 -> Add/2
  Constant1/1 -> Add/1
  Constant2/1 -> Add1/1
  In2/1 -> Add1/2
  Add1/1 -> Mux/2
  Constant3/1 -> Add2/1
  In3/1 -> Add2/2
  Add2/1 -> Mux/3
  Mux/1 -> MATLAB Function/2(u)

== system Simulacion_Estrategias/PTO DE EQUILIBRIO LQR CON MODELO LINEAL Y NO LIENAL/Subsystem1 ==
  In1 : Inport
  In2 : Inport  Port=2
  In3 : Inport  Port=3
  Add : Sum
  Add1 : Sum
  Add2 : Sum
  Constant : Constant  Value=[x10; x20; x30]
  Constant1 : Constant  Value=u10
  Constant2 : Constant  Value=u20
  Constant3 : Constant  Value=u30
  Gain : Gain  Gain=CL  Multiplication=Matrix(K*u)
  Integrator : Integrator  InitialCondition=[x10; x20; x30]+xini1
  MATLAB Function : MATLAB Function  TreatAsAtomicUnit=on
  Mux : Mux  Inputs=3
  Subtract : Sum  Inputs=+-
  Out1 : Outport
  Estados : Outport  Port=2
  wires:
  Mux/1 -> MATLAB Function/2(u)
  Add2/1 -> Mux/3
  In3/1 -> Add2/2
  Constant3/1 -> Add2/1
  Add1/1 -> Mux/2
  In2/1 -> Add1/2
  Constant2/1 -> Add1/1
  Constant1/1 -> Add/1
  In1/1 -> Add/2
  Add/1 -> Mux/1
  MATLAB Function/1(F) -> Integrator/1
  Gain/1 -> Out1/1
  Subtract/1 -> Gain/1, Estados/1
  Constant/1 -> Subtract/2
  Integrator/1 -> Subtract/1, MATLAB Function/1(x)

== matlab function Simulacion_Estrategias/POLOS COMPLEJOS CON MODELO LINEAL Y NO LIENAL /Subsystem/MATLAB Function ==
  data: x input; u input; F output
function F = modelo_no_lineal(x,u)
%estados
x1 = x(1);
x2 = x(2);
x3 = x(3);
%entradas
u1 = u(1);
u2 = u(2);
u3 = u(3);
%parametros
a=3
b=4
c=2
d=9
e=4
f=5
g=2

f1 = x2;
f2 = -b/a*x3*x2-c/a*x1+d/a*u1*u2;
f3 = f/e*u3-g/e*x3*u2;
F = [f1; f2; f3];

== matlab function Simulacion_Estrategias/COMPARACION PID & PC CON MODELO NO LINEAL/Subsystem/MATLAB Function ==
  data: x input; u input; F output
function F = modelo_no_lineal(x,u)
%estados
x1 = x(1);
x2 = x(2);
x3 = x(3);
%entradas
u1 = u(1);
u2 = u(2);
u3 = u(3);
%parametros
a=3
b=4
c=2
d=9
e=4
f=5
g=2

f1 = x2;
f2 = -b/a*x3*x2-c/a*x1+d/a*u1*u2;
f3 = f/e*u3-g/e*x3*u2;
F = [f1; f2; f3];

== matlab function Simulacion_Estrategias/1DOF1 CON MODELO LINEAL Y NO LIENAL/Subsystem/MATLAB Function ==
  data: x input; u input; F output
function F = modelo_no_lineal(x,u)
%estados
x1 = x(1);
x2 = x(2);
x3 = x(3);
%entradas
u1 = u(1);
u2 = u(2);
u3 = u(3);
%parametros
a=3
b=4
c=2
d=9
e=4
f=5
g=2

f1 = x2;
f2 = -b/a*x3*x2-c/a*x1+d/a*u1*u2;
f3 = f/e*u3-g/e*x3*u2;
F = [f1; f2; f3];

== matlab function Simulacion_Estrategias/COMPARACION PID & PC CON MODELO NO LINEAL/Subsystem1/MATLAB Function ==
  data: x input; u input; F output
function F = modelo_no_lineal(x,u)
%estados
x1 = x(1);
x2 = x(2);
x3 = x(3);
%entradas
u1 = u(1);
u2 = u(2);
u3 = u(3);
%parametros
a=3
b=4
c=2
d=9
e=4
f=5
g=2

f1 = x2;
f2 = -b/a*x3*x2-c/a*x1+d/a*u1*u2;
f3 = f/e*u3-g/e*x3*u2;
F = [f1; f2; f3];

== matlab function Simulacion_Estrategias/COMPARACION PID Y LQR CON MODELO NO LINEAL/Subsystem1/MATLAB Function ==
  data: x input; u input; F output
function F = modelo_no_lineal(x,u)
%estados
x1 = x(1);
x2 = x(2);
x3 = x(3);
%entradas
u1 = u(1);
u2 = u(2);
u3 = u(3);
%parametros
a=3
b=4
c=2
d=9
e=4
f=5
g=2

f1 = x2;
f2 = -b/a*x3*x2-c/a*x1+d/a*u1*u2;
f3 = f/e*u3-g/e*x3*u2;
F = [f1; f2; f3];

== matlab function Simulacion_Estrategias/COMPARACION PID Y LQR CON MODELO NO LINEAL/Subsystem/MATLAB Function ==
  data: x input; u input; F output
function F = modelo_no_lineal(x,u)
%estados
x1 = x(1);
x2 = x(2);
x3 = x(3);
%entradas
u1 = u(1);
u2 = u(2);
u3 = u(3);
%parametros
a=3
b=4
c=2
d=9
e=4
f=5
g=2

f1 = x2;
f2 = -b/a*x3*x2-c/a*x1+d/a*u1*u2;
f3 = f/e*u3-g/e*x3*u2;
F = [f1; f2; f3];

== matlab function Simulacion_Estrategias/1DOF PUNTO 6 CON MODELO LINEAL Y NO LIENAL/Subsystem/MATLAB Function ==
  data: x input; u input; F output
function F = modelo_no_lineal(x,u)
%estados
x1 = x(1);
x2 = x(2);
x3 = x(3);
%entradas
u1 = u(1);
u2 = u(2);
u3 = u(3);
%parametros
a=3
b=4
c=2
d=9
e=4
f=5
g=2

f1 = x2;
f2 = -b/a*x3*x2-c/a*x1+d/a*u1*u2;
f3 = f/e*u3-g/e*x3*u2;
F = [f1; f2; f3];

== matlab function Simulacion_Estrategias/PTO DE EQUILIBRIO LQR CON MODELO LINEAL Y NO LIENAL/Subsystem1/MATLAB Function ==
  data: x input; u input; F output
function F = modelo_no_lineal(x,u)
%estados
x1 = x(1);
x2 = x(2);
x3 = x(3);
%entradas
u1 = u(1);
u2 = u(2);
u3 = u(3);
%parametros
a=3
b=4
c=2
d=9
e=4
f=5
g=2

f1 = x2;
f2 = -b/a*x3*x2-c/a*x1+d/a*u1*u2;
f3 = f/e*u3-g/e*x3*u2;
F = [f1; f2; f3];
